simulink model "A_BPSK_ruido"  (Simulink 8.3)
settings: Solver=VariableStepDiscrete  StartTime=0.0  StopTime=sim_t  RelTol=1e-3
undefined symbols (not defined in the file): A1b, A3b, BSTb, PZb, STb
libraries: commrandsrc2 x1, dsparch4 x1
settings Model: Creator=usuario  LastModifiedBy=C.JO2COR
settings OptimizationCC: ExpressionDepthLimit=2147483647  InitFltsAndDblsToZero=on
settings DebuggingCC: SaveWithParameterizedLinksMsg=none  SignalResolutionControl=TryResolveAllWithWarning  MultiTaskDSMMsg=warning  MultiTaskCondExecSysMsg=none  FrameProcessingCompatibilityMsg=error
settings GRTTargetCC: TargetFcnLib=ansi_tfl_tmw.mat
settings ConfigComp: CovMetricSettings=dw  CovHtmlReporting=on  CovSaveCumulativeToWorkspaceVar=on  CovSaveSingleToWorkspaceVar=on  CovExternalEMLEnable=off  CovSFcnEnable=off

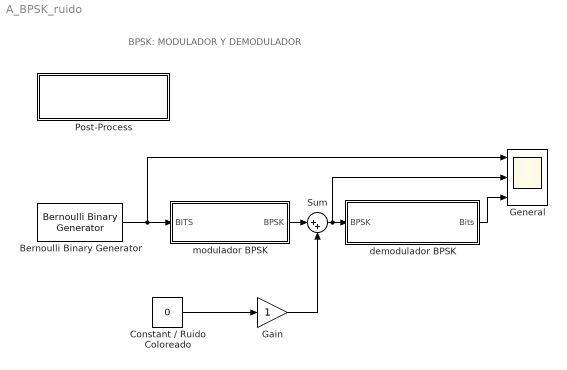
== system A_BPSK_ruido ==
  note: BPSK: MODULADOR Y DEMODULADOR
  Bernoulli Binary Generator : commrandsrc2/Bernoulli Binary Generator  P=PZb  seed=51  Ts=BSTb  frameBased=off  sampPerFrame=1  orient=off  outDataType=double
  Constant / Ruido Coloreado : Constant  Value=0
  Gain : Gain
  General : Scope  NumInputPorts=3
      settings: YMin=-5~-5~-5  YMax=5~5~5
  Post-Process : Subsystem  mask{sim_t=100, BSTb=5, FFb=1, A1b=0.4}
      mask prompts: sim_t "Sim Time [100]"; BSTb "Source Sample Time"; FFb "Freq. factor [1]"; A1b "Mod - Amp Sine [2]"
      mask init:
      | %sim_t = 100; %simulation time
      | %BSTb = 5; % source sample time
      | PZb = .4; % probability of zero
      | %STb = 1/20; % sample time
      | %SxPb = 50; % samples per period
      | %A1b = 2; % amplitude sine 1 - mod.
      | %A2b = .5; % amplitude sine 2 - mod.
      | A3b = 1; % amplitude sine 3 - demod.
      | 
      | switch sim_t
      |     case 1
      |         sim_t = 50;
      |     case 2
      |         sim_t = 100;
      |     case 3
      |         sim_t = 250;
      |     case 4
      |         sim_t = 500;
      |     case 5
      |         sim_t = 1000;        
      | end
      | 
      | % Sample Time Source Configure
      | switch BSTb
      |     case 1
      |         BSTb = 3;
      |     case 2
      |         BSTb = 5;
      |     case 3
      |         BSTb = 8;
      |     case 4
      |         BSTb = 10;
      |     case 5
      |         BST = 12;        
      | end
      | 
      | STb=(1/BSTb*1/4)*1/FFb;
      | %SxP=50*1/FF;
      | SxPb=(BSTb*10);
      | 
      | assignin('base','sim_t', sim_t );
      | assignin('base','FFb', FFb );
      | assignin('base','BSTb', BSTb );
      | assignin('base','PZb', PZb );
      | assignin('base','STb', STb );
      | assignin('base','SxPb', SxPb );
      | assignin('base','A1b', A1b );
      | %assignin('base','A2b', A2b );
      | assignin('base','A3b', A3b );
      mask TypeOptions sim_t: 50 | 100 | 250 | 500 | 1000
      mask TypeOptions BSTb: 3 | 5 | 8 | 10 | 12
      mask Display: disp('Sim Parameters')
  Sum : Sum  Inputs=|++
  demodulador BPSK : Subsystem
  modulador BPSK : Subsystem
  wires:
  Bernoulli Binary Generator/1 -> modulador BPSK/1(BITS), General/1
  demodulador BPSK/1(Bits) -> General/3
  Constant / Ruido Coloreado/1 -> Gain/1
  Gain/1 -> Sum/2
  modulador BPSK/1(BPSK) -> Sum/1
  Sum/1 -> General/2, demodulador BPSK/1(BPSK)

== system A_BPSK_ruido/Post-Process ==

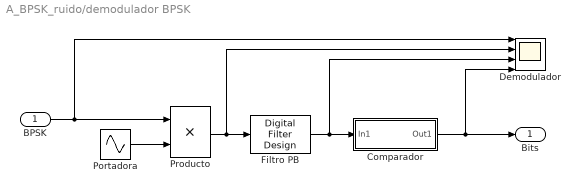
== system A_BPSK_ruido/demodulador BPSK ==
  BPSK : Inport
  Comparador : Subsystem
  Demodulador : Scope  NumInputPorts=4
  Filtro PB : dsparch4/Digital Filter Design  mwdsp_browser_bugfix_var=off
  Portadora : Sin  SineType=Sample based  Amplitude=A3b  Frequency=2*10*pi  Samples=SxPb  SampleTime=STb
  Producto : Product  RndMeth=Zero
  Bits : Outport
  wires:
  BPSK/1 -> Producto/1, Demodulador/1
  Portadora/1 -> Producto/2
  Producto/1 -> Filtro PB/1, Demodulador/2
  Filtro PB/1 -> Demodulador/3, Comparador/1(In1)
  Comparador/1(Out1) -> Bits/1, Demodulador/4

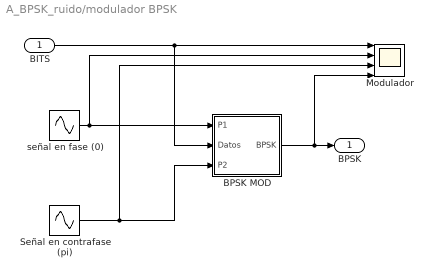
== system A_BPSK_ruido/modulador BPSK ==
  BITS : Inport
  BPSK MOD : Subsystem
  Modulador : Scope  NumInputPorts=4
      settings: YMin=-5~-5~-5~-5  YMax=5~5~5~5
  Señal en contrafase (pi) : Sin  SineType=Sample based  Amplitude=A1b  Frequency=2*10*pi  Phase=-pi  Samples=SxPb  SampleTime=STb  Offset=SxPb/2
  señal en fase (0) : Sin  SineType=Sample based  Amplitude=A1b  Frequency=2*10*pi  Samples=SxPb  SampleTime=STb
  BPSK : Outport
  wires:
  BITS/1 -> Modulador/1, BPSK MOD/2(Datos)
  señal en fase (0)/1 -> BPSK MOD/1(P1), Modulador/2
  Señal en contrafase (pi)/1 -> Modulador/3, BPSK MOD/3(P2)
  BPSK MOD/1(BPSK) -> Modulador/4, BPSK/1

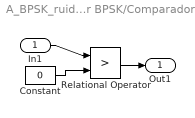
== system A_BPSK_ruido/demodulador BPSK/Comparador ==
  In1 : Inport
  Constant : Constant  Value=0
  Relational Operator : RelationalOperator  Operator=>  OutDataTypeStr=boolean
  Out1 : Outport
  wires:
  Constant/1 -> Relational Operator/2
  In1/1 -> Relational Operator/1
  Relational Operator/1 -> Out1/1

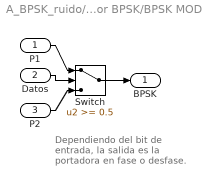
== system A_BPSK_ruido/modulador BPSK/BPSK MOD ==
  note: Dependiendo del bit
      | de entrada,
      | la salida es la portadora
      | en fase o desfase.
  P1 : Inport
  Datos : Inport  Port=2
  P2 : Inport  Port=3
  Switch : Switch  Threshold=0.5
  BPSK : Outport
  wires:
  P1/1 -> Switch/1
  Datos/1 -> Switch/2
  Switch/1 -> BPSK/1
  P2/1 -> Switch/3
